simulink model "zad2_model"  (R2018a)
settings: Solver=VariableStepAuto  StartTime=0.0  StopTime=10.0  RelTol=1e-3
values from neighbouring files (symbols this model uses):
  a = 500    [zad2.m]
  c = 400    [zad1.m]    (also in zad2.m)
  F = 1000    [zad2.m]
  M = 1000    [zad1.m]    (also in zad2.m)
settings Model: Creator=student  LastModifiedBy=student

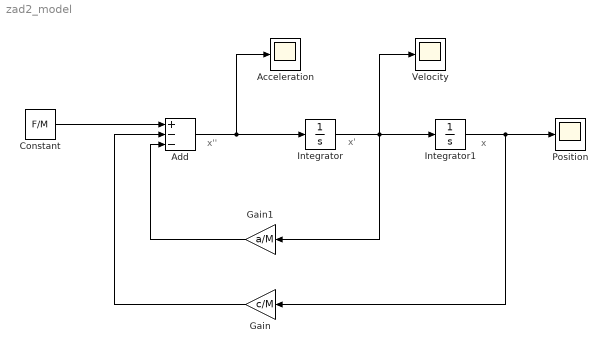
== system zad2_model ==
  note: x'
  note: x''
  note: x
  "Acceleration " : Scope
  Add : Sum  Inputs=+--
  Constant : Constant  Value=F/M
  Gain : Gain  Gain=c/M
  Gain1 : Gain  Gain=a/M
  Integrator : Integrator
  Integrator1 : Integrator
  "Position " : Scope
  "Velocity " : Scope
  wires:
  Add/1 -> "Acceleration "/1, Integrator/1
  Integrator/1 -> "Velocity "/1, Gain1/1, Integrator1/1
  Gain1/1 -> Add/3
  Integrator1/1 -> "Position "/1, Gain/1
  Gain/1 -> Add/2
  Constant/1 -> Add/1
